simulink model "fs"  (Simulink 7.6)
settings: Solver=ode45  StartTime=0.0  StopTime=10.0  MaxStep=1e-2  RelTol=1e-3
settings Model: Creator=John  LastModifiedBy=John
settings DebuggingCC: SolverPrmCheckMsg=none

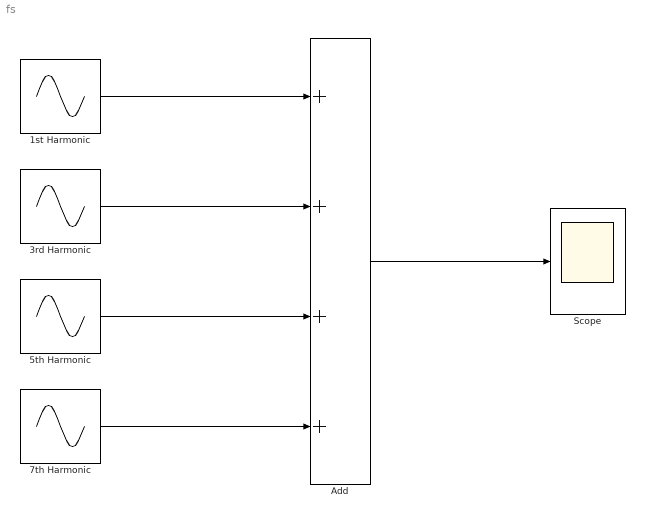
== system fs ==
  1st Harmonic : Sin  Frequency=pi  Phase=-pi/2  SampleTime=0
  3rd Harmonic : Sin  Amplitude=1/3  Frequency=3*pi  Phase=pi/2  SampleTime=0
  5th Harmonic : Sin  Amplitude=1/5  Frequency=5*pi  Phase=-pi/2  SampleTime=0
  7th Harmonic : Sin  Amplitude=1/7  Frequency=7*pi  Phase=pi/2  SampleTime=0
  Add : Sum  Inputs=++++
  Scope : Scope
  wires:
  1st Harmonic/1 -> Add/1
  3rd Harmonic/1 -> Add/2
  5th Harmonic/1 -> Add/3
  7th Harmonic/1 -> Add/4
  Add/1 -> Scope/1
